simulink model "AccelCtrl_ACC"  (Simulink 8.5)
settings: Solver=ode45  StartTime=0.0  StopTime=inf  RelTol=1e-3
values from neighbouring files (symbols this model uses):
  m = 336.83    [makeBikeModel.m]    (also in makePlants.m)
libraries: CarMaker4SL x33, simulink x2
(part 2 of 2)

== system AccelCtrl_ACC/CarMaker/IPG Vehicle/CarAndTrailer/Forces/Vehicle Forces ==
  Sync_In : Inport
  Bus Creator1 : BusCreator  Inputs=12
  Bus Creator8 : BusCreator  Inputs=16
  BusCreator1 : BusCreator
  BusCreator2 : BusCreator  Inputs=9
  Demux : Demux  Outputs=16
  Demux1 : Demux  Outputs=12
  Demux2 : Demux  Outputs=13
  Forces : S-Function  FunctionName=CM_Sfun  Parameters='Forces'
  Terminator : Terminator
  Sync_Out : Outport
  Car.Virtual : Outport  Port=2
  Car.Aero : Outport  Port=3
  Car.Load : Outport  Port=4
  wires:
  BusCreator1/1 -> Terminator/1  "Aero IF (in)"
  Demux2/13 -> BusCreator2/9  "car Aero Trq_1 z"
  Demux2/12 -> BusCreator2/8  "car Aero Trq_1 y"
  Demux2/11 -> BusCreator2/7  "car Aero Trq_1 x"
  Demux2/10 -> BusCreator2/6  "car Aero Frc_1 z"
  Demux2/9 -> BusCreator2/5  "car Aero Frc_1 y"
  Demux2/8 -> BusCreator2/4  "car Aero Frc_1 x"
  Demux2/7 -> BusCreator2/3  "car Aero PoA_1 z"
  Demux2/6 -> BusCreator2/2  "car Aero PoA_1 y"
  Demux2/5 -> BusCreator2/1  "car Aero PoA_1 x"
  Demux2/4 -> BusCreator1/4  "car Aero tau_1"
  Demux2/3 -> BusCreator1/3  "car Aero ApproachVel_1 z"
  Demux2/2 -> BusCreator1/2  "car Aero ApproachVel_1 y"
  Demux2/1 -> BusCreator1/1  "car Aero ApproachVel_1 x"
  Demux/16 -> Bus Creator8/16  "Car Load_3 tz"
  Demux/15 -> Bus Creator8/15  "Car Load_3 ty"
  Demux/14 -> Bus Creator8/14  "Car Load_3 tx"
  Demux/13 -> Bus Creator8/13  "Car Load_3 mass"
  Demux1/12 -> Bus Creator1/12  "Car Virtual Trq_0 z"
  Demux1/11 -> Bus Creator1/11  "Car Virtual Trq_0 y"
  Demux1/10 -> Bus Creator1/10  "Car Virtual Trq_0 x"
  Demux1/9 -> Bus Creator1/9  "Car Virtual Trq_1 z"
  Demux1/8 -> Bus Creator1/8  "Car Virtual Trq_1 y"
  Demux1/7 -> Bus Creator1/7  "Car Virtual Trq_1 x"
  Demux1/6 -> Bus Creator1/6  "Car Virtual Frc_0 z"
  Demux1/5 -> Bus Creator1/5  "Car Virtual Frc_0 y"
  Demux1/4 -> Bus Creator1/4  "Car Virtual Frc_0 x"
  Sync_In/1 -> Forces/1
  Forces/1 -> Sync_Out/1
  BusCreator2/1 -> Car.Aero/1
  Demux1/1 -> Bus Creator1/1  "Car Virtual Frc_1 x"
  Demux1/2 -> Bus Creator1/2  "Car Virtual Frc_1 y"
  Demux1/3 -> Bus Creator1/3  "Car Virtual Frc_1 z"
  Forces/3 -> Demux2/1
  Forces/2 -> Demux1/1
  Bus Creator1/1 -> Car.Virtual/1
  Bus Creator8/1 -> Car.Load/1
  Demux/1 -> Bus Creator8/1  "Car Load_0 mass"
  Demux/2 -> Bus Creator8/2  "Car Load_0 tx"
  Demux/3 -> Bus Creator8/3  "Car Load_0 ty"
  Demux/4 -> Bus Creator8/4  "Car Load_0 tz"
  Demux/5 -> Bus Creator8/5  "Car Load_1 mass"
  Demux/6 -> Bus Creator8/6  "Car Load_1 tx"
  Demux/7 -> Bus Creator8/7  "Car Load_1 ty"
  Demux/8 -> Bus Creator8/8  "Car Load_1 tz"
  Demux/9 -> Bus Creator8/9  "Car Load_2 mass"
  Demux/10 -> Bus Creator8/10  "Car Load_2 tx"
  Demux/11 -> Bus Creator8/11  "Car Load_2 ty"
  Demux/12 -> Bus Creator8/12  "Car Load_2 tz"
  Forces/4 -> Demux/1

== system AccelCtrl_ACC/CarMaker/IPG Vehicle/CarAndTrailer/Trailer/CreateBus Car.Hitch.FrcTrq ==
  In1 : Inport
  Bus Creator7 : BusCreator  Inputs=6
  Demux7 : Demux  Outputs=6
  Out1 : Outport
  wires:
  In1/1 -> Demux7/1
  Bus Creator7/1 -> Out1/1
  Demux7/6 -> Bus Creator7/6  "Car Hitch Trq2Car z"
  Demux7/5 -> Bus Creator7/5  "Car Hitch Trq2Car y"
  Demux7/4 -> Bus Creator7/4  "Car Hitch Trq2Car x"
  Demux7/3 -> Bus Creator7/3  "Car Hitch Frc2Car z"
  Demux7/2 -> Bus Creator7/2  "Car Hitch Frc2Car y"
  Demux7/1 -> Bus Creator7/1  "Car Hitch Frc2Car x"

== system AccelCtrl_ACC/CarMaker/IPG Vehicle/CarAndTrailer/Trailer/CreateBus Vhcl.Motion ==
  In1 : Inport
  BusCreator : BusCreator  Inputs=15
  Demux : Demux  Outputs=15
  Out1 : Outport
  wires:
  Demux/15 -> BusCreator/15  "Vhcl YawAcc"
  Demux/14 -> BusCreator/14  "Vhcl YawVel"
  Demux/13 -> BusCreator/13  "Vhcl Yaw"
  Demux/12 -> BusCreator/12  "Vhcl PitchAcc"
  Demux/11 -> BusCreator/11  "Vhcl PitchVel"
  Demux/10 -> BusCreator/10  "Vhcl Pitch"
  Demux/9 -> BusCreator/9  "Vhcl RollAcc"
  Demux/8 -> BusCreator/8  "Vhcl RollVel"
  Demux/7 -> BusCreator/7  "Vhcl Roll"
  Demux/6 -> BusCreator/6  "Vhcl Hitch_Pos z"
  Demux/5 -> BusCreator/5  "Vhcl Hitch_Pos y"
  Demux/4 -> BusCreator/4  "Vhcl Hitch_Pos x"
  Demux/3 -> BusCreator/3  "Vhcl sRoad"
  Demux/2 -> BusCreator/2  "Vhcl Distance"
  Demux/1 -> BusCreator/1  "Vhcl v"
  In1/1 -> Demux/1
  BusCreator/1 -> Out1/1

== system AccelCtrl_ACC/CarMaker/IPG Vehicle/CarAndTrailer/Trailer/CreateBus Vhcl.PoI ==
  In1 : Inport
  Bus Creator3 : BusCreator  Inputs=18
  Demux3 : Demux  Outputs=18
  Out1 : Outport
  wires:
  Demux3/18 -> Bus Creator3/18  "Vhcl PoI_GCS Elev"
  Demux3/17 -> Bus Creator3/17  "Vhcl PoI_GCS Lat"
  Demux3/16 -> Bus Creator3/16  "Vhcl PoI_GCS Long"
  Demux3/15 -> Bus Creator3/15  "Vhcl PoI_Acc_1 z"
  Demux3/14 -> Bus Creator3/14  "Vhcl PoI_Acc_1 y"
  Demux3/13 -> Bus Creator3/13  "Vhcl PoI_Acc_1 x"
  Demux3/12 -> Bus Creator3/12  "Vhcl PoI_Vel_1 z"
  Demux3/11 -> Bus Creator3/11  "Vhcl PoI_Vel_1 y"
  Demux3/10 -> Bus Creator3/10  "Vhcl PoI_Vel_1 x"
  Demux3/9 -> Bus Creator3/9  "Vhcl PoI_Acc z"
  Demux3/8 -> Bus Creator3/8  "Vhcl PoI_Acc y"
  Demux3/7 -> Bus Creator3/7  "Vhcl PoI_Acc x"
  Demux3/6 -> Bus Creator3/6  "Vhcl PoI_Vel z"
  Demux3/5 -> Bus Creator3/5  "Vhcl PoI_Vel y"
  Demux3/4 -> Bus Creator3/4  "Vhcl PoI_Vel x"
  Demux3/3 -> Bus Creator3/3  "Vhcl PoI_Pos z"
  Demux3/2 -> Bus Creator3/2  "Vhcl PoI_Pos y"
  In1/1 -> Demux3/1
  Bus Creator3/1 -> Out1/1
  Demux3/1 -> Bus Creator3/1  "Vhcl PoI_Pos x"

== system AccelCtrl_ACC/CarMaker/IPG Vehicle/CarAndTrailer/Trailer/CreateBus Vhcl.Steering ==
  In1 : Inport
  Bus Creator3 : BusCreator
  Demux : Demux
  Out1 : Outport
  wires:
  Bus Creator3/1 -> Out1/1
  Demux/1 -> Bus Creator3/1  "Vhcl Steering Ang"
  Demux/3 -> Bus Creator3/3  "Vhcl Steering AngAcc"
  Demux/2 -> Bus Creator3/2  "Vhcl Steering AngVel"
  Demux/4 -> Bus Creator3/4  "Vhcl Steering Trq"
  In1/1 -> Demux/1

== system AccelCtrl_ACC/CarMaker/IPG Vehicle/CarAndTrailer/Trailer/CreateBus Vhcl.Wheel.FL ==
  In1 : Inport
  Bus Creator3 : BusCreator  Inputs=14
  Demux3 : Demux  Outputs=14
  Out1 : Outport
  wires:
  Demux3/14 -> Bus Creator3/14  "Vhcl Wheel FL Trq_WhlBearing"
  Demux3/13 -> Bus Creator3/13  "Vhcl Wheel FL Trq_T2W"
  Demux3/12 -> Bus Creator3/12  "Vhcl Wheel FL SideSlip"
  Demux3/11 -> Bus Creator3/11  "Vhcl Wheel FL LongSlip"
  Demux3/10 -> Bus Creator3/10  "Vhcl Wheel FL vBelt"
  Demux3/9 -> Bus Creator3/9  "Vhcl Wheel FL Fz"
  Demux3/8 -> Bus Creator3/8  "Vhcl Wheel FL Fy"
  Demux3/7 -> Bus Creator3/7  "Vhcl Wheel FL Fx"
  Demux3/6 -> Bus Creator3/6  "Vhcl Wheel FL r_zxy z"
  Demux3/5 -> Bus Creator3/5  "Vhcl Wheel FL r_zxy y"
  Demux3/4 -> Bus Creator3/4  "Vhcl Wheel FL r_zxy x"
  Demux3/3 -> Bus Creator3/3  "Vhcl Wheel FL t z"
  Demux3/2 -> Bus Creator3/2  "Vhcl Wheel FL t y"
  In1/1 -> Demux3/1
  Bus Creator3/1 -> Out1/1
  Demux3/1 -> Bus Creator3/1  "Vhcl Wheel FL t x"

== system AccelCtrl_ACC/CarMaker/IPG Vehicle/CarAndTrailer/Trailer/CreateBus Vhcl.Wheel.FR ==
  In1 : Inport
  Bus Creator3 : BusCreator  Inputs=14
  Demux3 : Demux  Outputs=14
  Out1 : Outport
  wires:
  Demux3/14 -> Bus Creator3/14  "Vhcl Wheel FR Trq_WhlBearing"
  Demux3/13 -> Bus Creator3/13  "Vhcl Wheel FR Trq_T2W"
  Demux3/12 -> Bus Creator3/12  "Vhcl Wheel FR SideSlip"
  Demux3/11 -> Bus Creator3/11  "Vhcl Wheel FR LongSlip"
  Demux3/10 -> Bus Creator3/10  "Vhcl Wheel FR vBelt"
  Demux3/9 -> Bus Creator3/9  "Vhcl Wheel FR Fz"
  Demux3/8 -> Bus Creator3/8  "Vhcl Wheel FR Fy"
  Demux3/7 -> Bus Creator3/7  "Vhcl Wheel FR Fx"
  Demux3/6 -> Bus Creator3/6  "Vhcl Wheel FR r_zxy z"
  Demux3/5 -> Bus Creator3/5  "Vhcl Wheel FR r_zxy y"
  Demux3/4 -> Bus Creator3/4  "Vhcl Wheel FR r_zxy x"
  Demux3/3 -> Bus Creator3/3  "Vhcl Wheel FR t z"
  Demux3/2 -> Bus Creator3/2  "Vhcl Wheel FR t y"
  In1/1 -> Demux3/1
  Bus Creator3/1 -> Out1/1
  Demux3/1 -> Bus Creator3/1  "Vhcl Wheel FR t x"

== system AccelCtrl_ACC/CarMaker/IPG Vehicle/CarAndTrailer/Trailer/CreateBus Vhcl.Wheel.RL ==
  In1 : Inport
  Bus Creator3 : BusCreator  Inputs=14
  Demux3 : Demux  Outputs=14
  Out1 : Outport
  wires:
  Demux3/14 -> Bus Creator3/14  "Vhcl Wheel RL Trq_WhlBearing"
  Demux3/13 -> Bus Creator3/13  "Vhcl Wheel RL Trq_T2W"
  Demux3/12 -> Bus Creator3/12  "Vhcl Wheel RL SideSlip"
  Demux3/11 -> Bus Creator3/11  "Vhcl Wheel RL LongSlip"
  Demux3/10 -> Bus Creator3/10  "Vhcl Wheel RL vBelt"
  Demux3/9 -> Bus Creator3/9  "Vhcl Wheel RL Fz"
  Demux3/8 -> Bus Creator3/8  "Vhcl Wheel RL Fy"
  Demux3/7 -> Bus Creator3/7  "Vhcl Wheel RL Fx"
  Demux3/6 -> Bus Creator3/6  "Vhcl Wheel RL r_zxy z"
  Demux3/5 -> Bus Creator3/5  "Vhcl Wheel RL r_zxy y"
  Demux3/4 -> Bus Creator3/4  "Vhcl Wheel RL r_zxy x"
  Demux3/3 -> Bus Creator3/3  "Vhcl Wheel RL t z"
  Demux3/2 -> Bus Creator3/2  "Vhcl Wheel RL t y"
  In1/1 -> Demux3/1
  Bus Creator3/1 -> Out1/1
  Demux3/1 -> Bus Creator3/1  "Vhcl Wheel RL t x"

== system AccelCtrl_ACC/CarMaker/IPG Vehicle/CarAndTrailer/Trailer/CreateBus Vhcl.Wheel.RR ==
  In1 : Inport
  Bus Creator3 : BusCreator  Inputs=14
  Demux3 : Demux  Outputs=14
  Out1 : Outport
  wires:
  Demux3/14 -> Bus Creator3/14  "Vhcl Wheel RR Trq_WhlBearing"
  Demux3/13 -> Bus Creator3/13  "Vhcl Wheel RR Trq_T2W"
  Demux3/12 -> Bus Creator3/12  "Vhcl Wheel RR SideSlip"
  Demux3/11 -> Bus Creator3/11  "Vhcl Wheel RR LongSlip"
  Demux3/10 -> Bus Creator3/10  "Vhcl Wheel RR vBelt"
  Demux3/9 -> Bus Creator3/9  "Vhcl Wheel RR Fz"
  Demux3/8 -> Bus Creator3/8  "Vhcl Wheel RR Fy"
  Demux3/7 -> Bus Creator3/7  "Vhcl Wheel RR Fx"
  Demux3/6 -> Bus Creator3/6  "Vhcl Wheel RR r_zxy z"
  Demux3/5 -> Bus Creator3/5  "Vhcl Wheel RR r_zxy y"
  Demux3/4 -> Bus Creator3/4  "Vhcl Wheel RR r_zxy x"
  Demux3/3 -> Bus Creator3/3  "Vhcl Wheel RR t z"
  Demux3/2 -> Bus Creator3/2  "Vhcl Wheel RR t y"
  In1/1 -> Demux3/1
  Bus Creator3/1 -> Out1/1
  Demux3/1 -> Bus Creator3/1  "Vhcl Wheel RR t x"

== system AccelCtrl_ACC/CarMaker/VehicleControl/AccelCtrl/ACC ECU/ACC Control ==
  ACC enabled : Inport
  Target Dtct : Inport  Port=2
  Target.ds : Inport  Port=3
  Target.dv : Inport  Port=4
  Desired time gap : Inport  Port=5
  Desired speed : Inport  Port=6
  Ax is NOTSET : Constant  Value=-99999
  Desired Distance Calculation with time gap : Subsystem  TreatAsAtomicUnit=on
  Distance Control Algorithm : Subsystem  TreatAsAtomicUnit=on
  Logical Operator : Logic  AllPortsSameDT=off
  Speed Control Algorithm : Subsystem  TreatAsAtomicUnit=on
  Target detected : simulink/Logic and Bit Operations/Compare To Zero  relop=>  OutDataTypeStr=uint8  ZeroCross=off
  desired Ax : Switch  Threshold=1  SaturateOnIntegerOverflow=on
  desired or NOTSET : Switch  Threshold=1  SaturateOnIntegerOverflow=on
  Desired Ax : Outport
  wires:
  Target.dv/1 -> Distance Control Algorithm/2(Target.dv[m/s]), Desired Distance Calculation with time gap/1(Target.dv)
  Target.ds/1 -> Distance Control Algorithm/1(Target.ds[m])
  Target Dtct/1 -> Target detected/1
  Distance Control Algorithm/1("  limited ax") -> desired Ax/1
  Target detected/1 -> desired Ax/2, Logical Operator/2
  Desired Distance Calculation with time gap/1(desired distance) -> Distance Control Algorithm/3(desired distance[m])
  Desired time gap/1 -> Desired Distance Calculation with time gap/2(desired time gap)
  Desired speed/1 -> Speed Control Algorithm/1(desire speed[m/s])
  Speed Control Algorithm/1(ax speed control) -> desired Ax/3, Distance Control Algorithm/4(ax speed control)
  ACC enabled/1 -> Logical Operator/1, desired or NOTSET/2
  Logical Operator/1 -> Desired Distance Calculation with time gap/Enable
  desired or NOTSET/1 -> Desired Ax/1
  desired Ax/1 -> desired or NOTSET/1
  Ax is NOTSET/1 -> desired or NOTSET/3

== system AccelCtrl_ACC/CarMaker/VehicleControl/AccelCtrl/ACC ECU/ACC User Input ==
  ACC Active ACC/Actual Speed : Switch  Threshold=1  SaturateOnIntegerOverflow=on
  Constant : Constant
  Init Desired time gap quantity : Subsystem  TreatAsAtomicUnit=on
  Is ACC enabled : CarMaker4SL/Read CM Dict  xname=AccelCtrl.ACC.IsActive  xsync=off
  Memory : Memory
  Read Car.v[m/s] : CarMaker4SL/Read CM Dict  xname=Car.v  xsync=off
  Read Init Velocity : CarMaker4SL/Read CM Parameter  xfile=Testrun  xkey=DrivMan.Init.Velocity  xnout=1  xdefaults=0  xmuxed=on
  Read Simulation Time : CarMaker4SL/Read CM Dict  xname=Time  xsync=off
  Read User desired speed : CarMaker4SL/Read CM Dict  xname=AccelCtrl.ACC.DesiredSpd  xsync=off
  Read User desired time gap : CarMaker4SL/Read CM Dict  xname=AccelCtrl.ACC.DesiredTGap  xsync=off
  Read init desired time gap from Inf : CarMaker4SL/Read CM Parameter  xfile=Vehicle  xkey=AccelCtrl.ACC.DesrTGap  xnout=1  xdefaults=1.8  xmuxed=off
  Switch : Switch  Criteria=u2 > Threshold
  Write desired speed : CarMaker4SL/Write CM Dict  xname=AccelCtrl.ACC.DesiredSpd  xsync=off
  kmh2ms : Gain  Gain=0.28
  ACC enabled : Outport
  Desired time gap[s] : Outport  Port=2
  Desired speed[m/s] : Outport  Port=3
  wires:
  Is ACC enabled/1 -> ACC enabled/1, ACC Active ACC/Actual Speed/2
  Read Car.v[m/s]/1 -> ACC Active ACC/Actual Speed/3
  ACC Active ACC/Actual Speed/1 -> Desired speed[m/s]/1, Write desired speed/1
  Read User desired time gap/1 -> Desired time gap[s]/1
  Constant/1 -> Memory/1
  Memory/1 -> Init Desired time gap quantity/Trigger
  Read init desired time gap from Inf/1 -> Init Desired time gap quantity/1("Init desired time gap ")
  Read Init Velocity/1 -> kmh2ms/1
  Switch/1 -> ACC Active ACC/Actual Speed/1
  Read User desired speed/1 -> Switch/1
  Read Simulation Time/1 -> Switch/2
  kmh2ms/1 -> Switch/3

== system AccelCtrl_ACC/CarMaker/VehicleControl/AccelCtrl/AccelCtrl/PI-Controller ==
  delta_ax : Inport
  DM_Gas : Inport  Port=2
  AxCtrl On : Inport  Port=3
  Add : Sum  SaturateOnIntegerOverflow=on  OutDataTypeStr=Inherit: Same as first input
  Integrator : Subsystem
  Read init i_gain from Inf : CarMaker4SL/Read CM Parameter  xfile=Vehicle  xkey=AccelCtrl.i_gain  xnout=1  xdefaults=0.001  xmuxed=off
  Read init p_gain from Inf : CarMaker4SL/Read CM Parameter  xfile=Vehicle  xkey=AccelCtrl.p_gain  xnout=1  xdefaults=0.001  xmuxed=off
  Saturation : Saturate  UpperLimit=1  LowerLimit=-1
  i_gain : Product  SaturateOnIntegerOverflow=on  OutDataTypeStr=Inherit: Same as first input
  p_gain : Product  SaturateOnIntegerOverflow=on  OutDataTypeStr=Inherit: Same as first input
  Gas or Brake : Outport
  wires:
  Saturation/1 -> Gas or Brake/1
  Add/1 -> Saturation/1
  p_gain/1 -> Add/1
  delta_ax/1 -> p_gain/2, i_gain/1
  i_gain/1 -> Integrator/1(I-Part)
  AxCtrl On/1 -> Integrator/2(AxCtrl On)
  DM_Gas/1 -> Integrator/3(Init I-part)
  Integrator/1("I-part tot ") -> Add/2
  Read init p_gain from Inf/1 -> p_gain/1
  Read init i_gain from Inf/1 -> i_gain/2

== system AccelCtrl_ACC/CarMaker/VehicleControl/AccelCtrl/AccelCtrl/controlled process variable  ==
  desired ax : Inport
  Read Car.ax : CarMaker4SL/Read CM Dict  xname=Car.ax  xsync=off
  Subtract : Sum  Inputs=+-  SaturateOnIntegerOverflow=on
  delta ax : Outport
  wires:
  desired ax/1 -> Subtract/1
  Read Car.ax/1 -> Subtract/2
  Subtract/1 -> delta ax/1

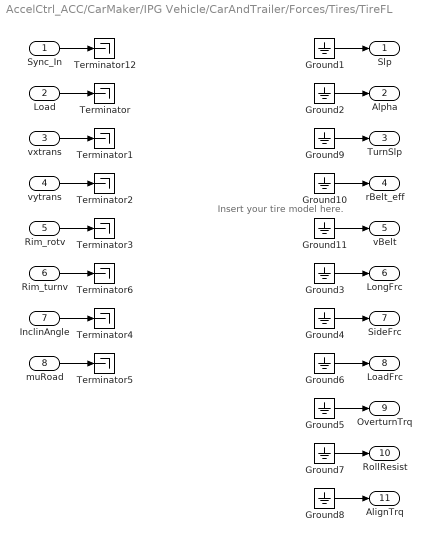
== system AccelCtrl_ACC/CarMaker/IPG Vehicle/CarAndTrailer/Forces/Tires/TireFL ==
  note: Insert your tire model here.
  Sync_In : Inport
  Load : Inport  Port=2
  vxtrans : Inport  Port=3
  vytrans : Inport  Port=4
  Rim_rotv : Inport  Port=5
  Rim_turnv : Inport  Port=6
  InclinAngle : Inport  Port=7
  muRoad : Inport  Port=8
  Ground{1..11} (11 alike) : Ground
  Terminator{,1..6,12} (8 alike) : Terminator
  Slp : Outport
  Alpha : Outport  Port=2
  TurnSlp : Outport  Port=3
  rBelt_eff : Outport  Port=4
  vBelt : Outport  Port=5
  LongFrc : Outport  Port=6
  SideFrc : Outport  Port=7
  LoadFrc : Outport  Port=8
  OverturnTrq : Outport  Port=9
  RollResist : Outport  Port=10
  AlignTrq : Outport  Port=11
  wires:
  Ground11/1 -> vBelt/1
  Ground10/1 -> rBelt_eff/1
  Ground9/1 -> TurnSlp/1
  Rim_turnv/1 -> Terminator6/1
  Sync_In/1 -> Terminator12/1
  Ground2/1 -> Alpha/1
  Ground3/1 -> LongFrc/1
  Ground4/1 -> SideFrc/1
  Ground5/1 -> OverturnTrq/1
  vxtrans/1 -> Terminator1/1
  vytrans/1 -> Terminator2/1
  Rim_rotv/1 -> Terminator3/1
  InclinAngle/1 -> Terminator4/1
  muRoad/1 -> Terminator5/1
  Load/1 -> Terminator/1
  Ground1/1 -> Slp/1
  Ground6/1 -> LoadFrc/1
  Ground7/1 -> RollResist/1
  Ground8/1 -> AlignTrq/1

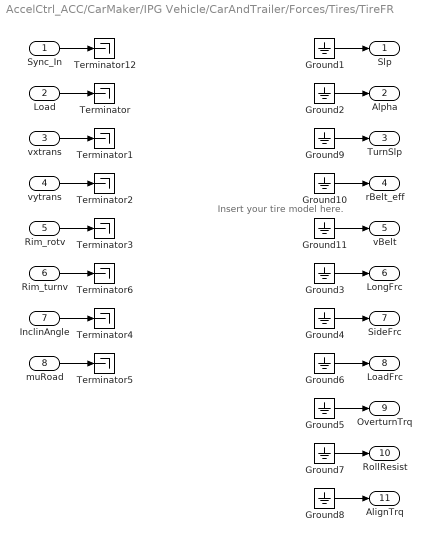
== system AccelCtrl_ACC/CarMaker/IPG Vehicle/CarAndTrailer/Forces/Tires/TireFR ==
  note: Insert your tire model here.
  Sync_In : Inport
  Load : Inport  Port=2
  vxtrans : Inport  Port=3
  vytrans : Inport  Port=4
  Rim_rotv : Inport  Port=5
  Rim_turnv : Inport  Port=6
  InclinAngle : Inport  Port=7
  muRoad : Inport  Port=8
  Ground{1..11} (11 alike) : Ground
  Terminator{,1..6,12} (8 alike) : Terminator
  Slp : Outport
  Alpha : Outport  Port=2
  TurnSlp : Outport  Port=3
  rBelt_eff : Outport  Port=4
  vBelt : Outport  Port=5
  LongFrc : Outport  Port=6
  SideFrc : Outport  Port=7
  LoadFrc : Outport  Port=8
  OverturnTrq : Outport  Port=9
  RollResist : Outport  Port=10
  AlignTrq : Outport  Port=11
  wires:
  Ground11/1 -> vBelt/1
  Ground10/1 -> rBelt_eff/1
  Ground9/1 -> TurnSlp/1
  Rim_turnv/1 -> Terminator6/1
  Sync_In/1 -> Terminator12/1
  Ground2/1 -> Alpha/1
  Ground3/1 -> LongFrc/1
  Ground4/1 -> SideFrc/1
  Ground5/1 -> OverturnTrq/1
  vxtrans/1 -> Terminator1/1
  vytrans/1 -> Terminator2/1
  Rim_rotv/1 -> Terminator3/1
  InclinAngle/1 -> Terminator4/1
  muRoad/1 -> Terminator5/1
  Load/1 -> Terminator/1
  Ground1/1 -> Slp/1
  Ground6/1 -> LoadFrc/1
  Ground7/1 -> RollResist/1
  Ground8/1 -> AlignTrq/1

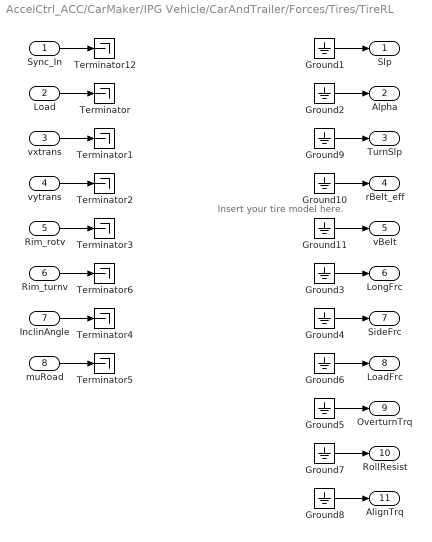
== system AccelCtrl_ACC/CarMaker/IPG Vehicle/CarAndTrailer/Forces/Tires/TireRL ==
  note: Insert your tire model here.
  Sync_In : Inport
  Load : Inport  Port=2
  vxtrans : Inport  Port=3
  vytrans : Inport  Port=4
  Rim_rotv : Inport  Port=5
  Rim_turnv : Inport  Port=6
  InclinAngle : Inport  Port=7
  muRoad : Inport  Port=8
  Ground{1..11} (11 alike) : Ground
  Terminator{,1..6,12} (8 alike) : Terminator
  Slp : Outport
  Alpha : Outport  Port=2
  TurnSlp : Outport  Port=3
  rBelt_eff : Outport  Port=4
  vBelt : Outport  Port=5
  LongFrc : Outport  Port=6
  SideFrc : Outport  Port=7
  LoadFrc : Outport  Port=8
  OverturnTrq : Outport  Port=9
  RollResist : Outport  Port=10
  AlignTrq : Outport  Port=11
  wires:
  Ground11/1 -> vBelt/1
  Ground10/1 -> rBelt_eff/1
  Ground9/1 -> TurnSlp/1
  Rim_turnv/1 -> Terminator6/1
  Sync_In/1 -> Terminator12/1
  Ground2/1 -> Alpha/1
  Ground3/1 -> LongFrc/1
  Ground4/1 -> SideFrc/1
  Ground5/1 -> OverturnTrq/1
  vxtrans/1 -> Terminator1/1
  vytrans/1 -> Terminator2/1
  Rim_rotv/1 -> Terminator3/1
  InclinAngle/1 -> Terminator4/1
  muRoad/1 -> Terminator5/1
  Load/1 -> Terminator/1
  Ground1/1 -> Slp/1
  Ground6/1 -> LoadFrc/1
  Ground7/1 -> RollResist/1
  Ground8/1 -> AlignTrq/1

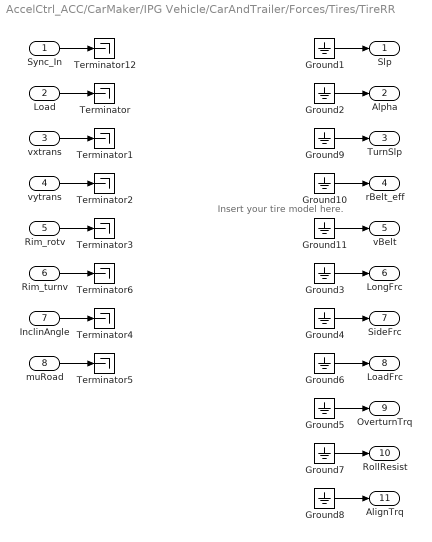
== system AccelCtrl_ACC/CarMaker/IPG Vehicle/CarAndTrailer/Forces/Tires/TireRR ==
  note: Insert your tire model here.
  Sync_In : Inport
  Load : Inport  Port=2
  vxtrans : Inport  Port=3
  vytrans : Inport  Port=4
  Rim_rotv : Inport  Port=5
  Rim_turnv : Inport  Port=6
  InclinAngle : Inport  Port=7
  muRoad : Inport  Port=8
  Ground{1..11} (11 alike) : Ground
  Terminator{,1..6,12} (8 alike) : Terminator
  Slp : Outport
  Alpha : Outport  Port=2
  TurnSlp : Outport  Port=3
  rBelt_eff : Outport  Port=4
  vBelt : Outport  Port=5
  LongFrc : Outport  Port=6
  SideFrc : Outport  Port=7
  LoadFrc : Outport  Port=8
  OverturnTrq : Outport  Port=9
  RollResist : Outport  Port=10
  AlignTrq : Outport  Port=11
  wires:
  Ground11/1 -> vBelt/1
  Ground10/1 -> rBelt_eff/1
  Ground9/1 -> TurnSlp/1
  Rim_turnv/1 -> Terminator6/1
  Sync_In/1 -> Terminator12/1
  Ground2/1 -> Alpha/1
  Ground3/1 -> LongFrc/1
  Ground4/1 -> SideFrc/1
  Ground5/1 -> OverturnTrq/1
  vxtrans/1 -> Terminator1/1
  vytrans/1 -> Terminator2/1
  Rim_rotv/1 -> Terminator3/1
  InclinAngle/1 -> Terminator4/1
  muRoad/1 -> Terminator5/1
  Load/1 -> Terminator/1
  Ground1/1 -> Slp/1
  Ground6/1 -> LoadFrc/1
  Ground7/1 -> RollResist/1
  Ground8/1 -> AlignTrq/1

== system AccelCtrl_ACC/CarMaker/VehicleControl/AccelCtrl/ACC ECU/ACC Control/Desired Distance Calculation with time gap ==
  Target.dv : Inport
  desired time gap : Inport  Port=2
  Enable : EnablePort
  Add : Sum  SaturateOnIntegerOverflow=on  OutDataTypeStr=Inherit: Same as first input
  MinMax : MinMax  Function=max  Inputs=2  SaturateOnIntegerOverflow=on  InputSameDT=on
  Product : Product  SaturateOnIntegerOverflow=on  OutDataTypeStr=Inherit: Same as first input
  Read Car.v[m/s] : CarMaker4SL/Read CM Dict  xname=Car.v  xsync=off
  Read init min distance from Inf : CarMaker4SL/Read CM Parameter  xfile=Vehicle  xkey=AccelCtrl.ACC.DistMin  xnout=1  xdefaults=20  xmuxed=off
  Write desired distance : CarMaker4SL/Write CM Dict  xname=AccelCtrl.ACC.DesiredDist  xsync=off
  desired distance : Outport  InitialOutput=0
  wires:
  Read Car.v[m/s]/1 -> Add/2
  Product/1 -> MinMax/1
  Add/1 -> Product/2
  desired time gap/1 -> Product/1
  Target.dv/1 -> Add/1
  MinMax/1 -> desired distance/1, Write desired distance/1
  Read init min distance from Inf/1 -> MinMax/2

== system AccelCtrl_ACC/CarMaker/VehicleControl/AccelCtrl/ACC ECU/ACC Control/Distance Control Algorithm ==
  Target.ds[m] : Inport
  Target.dv[m/s] : Inport  Port=2
  desired distance[m] : Inport  Port=3
  ax speed control : Inport  Port=4
  -2.5<=ax<=1 : Saturate  UpperLimit=1  LowerLimit=-2.5
  desired ax : Subsystem
  "  limited ax" : Outport  InitialOutput=0
  wires:
  ax speed control/1 -> desired ax/4(ax speed control)
  desired distance[m]/1 -> desired ax/3(desired distance[m])
  Target.dv[m/s]/1 -> desired ax/2(Target.dv[m/s])
  Target.ds[m]/1 -> desired ax/1(Target.ds[m])
  -2.5<=ax<=1/1 -> "  limited ax"/1
  desired ax/1(desired ax) -> -2.5<=ax<=1/1

== system AccelCtrl_ACC/CarMaker/VehicleControl/AccelCtrl/ACC ECU/ACC Control/Speed Control Algorithm ==
  desire speed[m/s] : Inport
  -0.35<=ax<=1 : Saturate  UpperLimit=1  LowerLimit=-0.35
  desired ax : Subsystem
  ax speed control : Outport  InitialOutput=0
  wires:
  desire speed[m/s]/1 -> desired ax/1(desire speed[m/s])
  desired ax/1(desired ax) -> -0.35<=ax<=1/1
  -0.35<=ax<=1/1 -> ax speed control/1

== system AccelCtrl_ACC/CarMaker/VehicleControl/AccelCtrl/ACC ECU/ACC User Input/Init Desired time gap quantity ==
  "Init desired time gap " : Inport
  Trigger : TriggerPort
  Write init time gap : CarMaker4SL/Write CM Dict  xname=AccelCtrl.ACC.DesiredTGap  xsync=off
  wires:
  "Init desired time gap "/1 -> Write init time gap/1

== system AccelCtrl_ACC/CarMaker/VehicleControl/AccelCtrl/AccelCtrl/PI-Controller/Integrator ==
  I-Part : Inport
  AxCtrl On : Inport  Port=2
  Init I-part : Inport  Port=3
  Add1 : Sum  SaturateOnIntegerOverflow=on  OutDataTypeStr=Inherit: Same as first input
  Memory : Memory
  Saturation : Saturate  UpperLimit=1  LowerLimit=-1
  Switch Ax  Init I-Part : Switch  Threshold=1  SaturateOnIntegerOverflow=on
  "I-part tot " : Outport
  wires:
  Saturation/1 -> Memory/1
  Switch Ax  Init I-Part/1 -> Add1/2
  Add1/1 -> Saturation/1, "I-part tot "/1
  I-Part/1 -> Add1/1
  AxCtrl On/1 -> Switch Ax  Init I-Part/2
  Memory/1 -> Switch Ax  Init I-Part/1
  Init I-part/1 -> Switch Ax  Init I-Part/3

== system AccelCtrl_ACC/CarMaker/VehicleControl/AccelCtrl/ACC ECU/ACC Control/Distance Control Algorithm/desired ax ==
  note: desired ax = (target.ds-desired.distance)/(kd)+target.dv/kv
  note: delta_ds
  Target.ds[m] : Inport
  Target.dv[m/s] : Inport  Port=2
  desired distance[m] : Inport  Port=3
  ax speed control : Inport  Port=4
  Add : Sum  SaturateOnIntegerOverflow=on  OutDataTypeStr=Inherit: Same as first input
  Divide : Product  Inputs=*/  SaturateOnIntegerOverflow=on  OutDataTypeStr=Inherit: Same as first input
  Divide1 : Product  Inputs=*/  SaturateOnIntegerOverflow=on  OutDataTypeStr=Inherit: Same as first input
  MinMax : MinMax  Inputs=2  SaturateOnIntegerOverflow=on  InputSameDT=on
  Read init distctrl.kd from Inf : CarMaker4SL/Read CM Parameter  xfile=Vehicle  xkey=AccelCtrl.ACC.DistCtrl.kd  xnout=1  xdefaults=36  xmuxed=off
  Read init distctrl.kv from Inf1 : CarMaker4SL/Read CM Parameter  xfile=Vehicle  xkey=AccelCtrl.ACC.DistCtrl.kv  xnout=1  xdefaults=2  xmuxed=off
  Subtract : Sum  Inputs=+-  SaturateOnIntegerOverflow=on  OutDataTypeStr=Inherit: Same as first input
  desired ax : Outport
  wires:
  MinMax/1 -> desired ax/1
  ax speed control/1 -> MinMax/2
  Add/1 -> MinMax/1
  Divide1/1 -> Add/2
  Divide/1 -> Add/1
  Subtract/1 -> Divide/1
  desired distance[m]/1 -> Subtract/2
  Target.ds[m]/1 -> Subtract/1
  Target.dv[m/s]/1 -> Divide1/1
  Read init distctrl.kd from Inf/1 -> Divide/2
  Read init distctrl.kv from Inf1/1 -> Divide1/2

== system AccelCtrl_ACC/CarMaker/VehicleControl/AccelCtrl/ACC ECU/ACC Control/Speed Control Algorithm/desired ax ==
  desire speed[m/s] : Inport
  Divide : Product  Inputs=*/  SaturateOnIntegerOverflow=on  OutDataTypeStr=Inherit: Same as first input
  Read Car.v[m/s] : CarMaker4SL/Read CM Dict  xname=Car.v  xsync=off
  Read init spdctrl.kv from Inf : CarMaker4SL/Read CM Parameter  xfile=Vehicle  xkey=AccelCtrl.ACC.SpdCtrl.kv  xnout=1  xdefaults=13  xmuxed=off
  Sum : Sum  Inputs=|+-  SaturateOnIntegerOverflow=on  OutDataTypeStr=Inherit: Same as first input
  desired ax : Outport
  wires:
  Divide/1 -> desired ax/1
  desire speed[m/s]/1 -> Sum/1
  Read Car.v[m/s]/1 -> Sum/2
  Sum/1 -> Divide/1
  Read init spdctrl.kv from Inf/1 -> Divide/2
